simulink model "ingenuity_2023b"  (R2023b)
settings: Solver=VariableStepAuto  StartTime=0.0  StopTime=1000  FixedStep=0.001  RelTol=1e-3
values from neighbouring files (symbols this model uses):
  NACA2412 =     [CL_CD.mat]
undefined symbols (not defined in the file or in its folder): Actor, init
libraries: cstblocks x8, sim3dlib x7
settings Model: Creator=39351  LastModifiedBy=antor
settings OptimizationCC: ReuseModelBlockBuffer=off

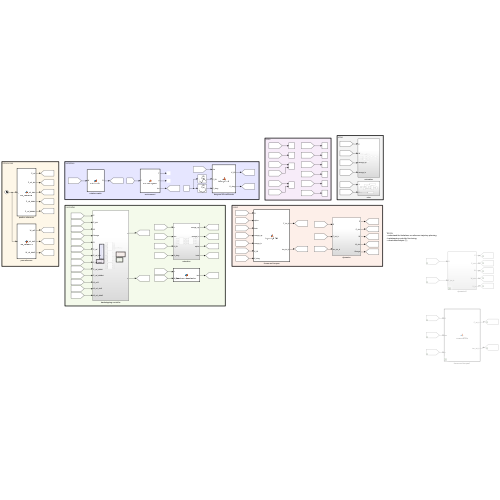
[thumbnail: Simulink's stored preview of the top-level diagram]
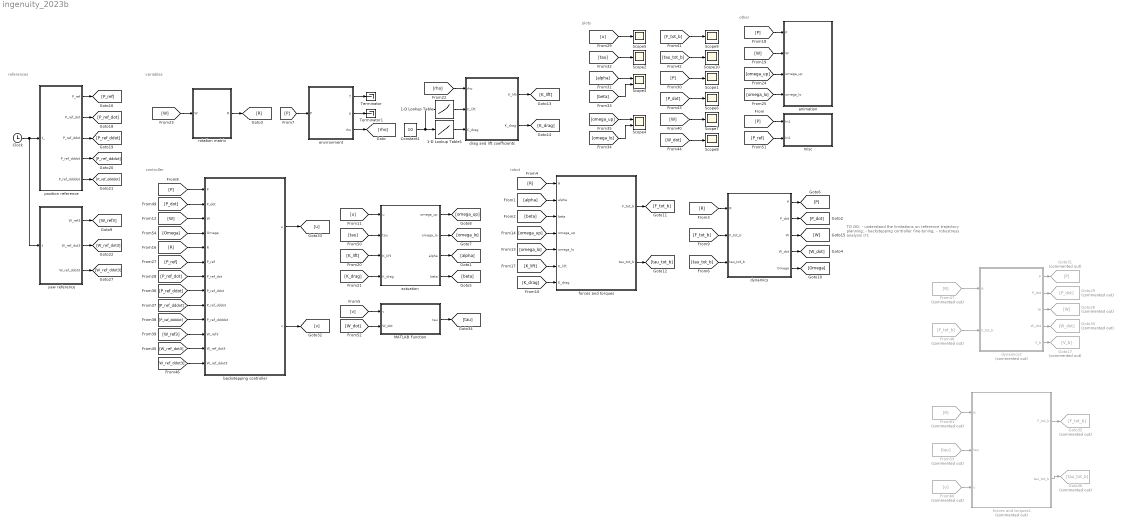
== system ingenuity_2023b ==
  note: TO DO:
      | - understand the limitations on reference trajectory planning;
      | - backstepping controller fine-tuning;
      | - robustness analysis (?);
  note: references
  note: other
  note: plots
  note: variables
  note: controller
  note: robot
  1-D Lookup Table : Lookup_n-D  NumberOfTableDimensions=1  BreakpointsForDimension1=NACA2412.CL(:,1)  Table=NACA2412.CL(:,2)  InternalRulePriority=Speed  RndMeth=Simplest
  1-D Lookup Table1 : Lookup_n-D  NumberOfTableDimensions=1  BreakpointsForDimension1=NACA2412.CD(:,1)  Table=NACA2412.CD(:,2)  InternalRulePriority=Speed  RndMeth=Simplest
  Clock : Clock
  Constant1 : Constant  Value=10
  From47 : From  Commented=on  GotoTag=R
  From48 : From  Commented=on  GotoTag=F_tot_b
  From53 : From  Commented=on  GotoTag=tau
  From60 : From  Commented=on  GotoTag=u
  From61 : From  Commented=on  GotoTag=R
  Goto17 : Goto  Commented=on  GotoTag=V_b
  Goto28 : Goto  Commented=on  GotoTag=W
  Goto29 : Goto  Commented=on  GotoTag=P_dot
  Goto30 : Goto  Commented=on  GotoTag=W_dot
  Goto31 : Goto  Commented=on  GotoTag=P
  Goto35 : Goto  Commented=on  GotoTag=F_tot_b
  Goto36 : Goto  Commented=on  GotoTag=tau_tot_b
  MATLAB Function : MATLAB Function  TreatAsAtomicUnit=on
  Scope{1..2,5..10} (8 alike) : Scope
  Scope3 : Scope  NumInputPorts=2
  Scope4 : Scope  NumInputPorts=2
  Terminator : Terminator
  Terminator1 : Terminator
  actuation : Subsystem
  animation : Subsystem
  backstepping controller : Subsystem
  drag and lift coefficients : MATLAB Function  TreatAsAtomicUnit=on
  dynamics : Subsystem
  dynamics2 : Subsystem  Commented=on
  environment : MATLAB Function  TreatAsAtomicUnit=on
  forces and torques : MATLAB Function  TreatAsAtomicUnit=on
  forces and torques1 : MATLAB Function  Commented=on  TreatAsAtomicUnit=on
  misc : Subsystem
  position reference : MATLAB Function  TreatAsAtomicUnit=on
  rotation matrix : MATLAB Function  TreatAsAtomicUnit=on
  yaw reference : MATLAB Function  TreatAsAtomicUnit=on
  wires:
  environment/1(T) -> Terminator/1
  environment/2(p) -> Terminator1/1
  environment/3(rho) -> [rho]
  [R] -> dynamics/1(R)
  dynamics/3(W) -> [W]
  [alpha] -> forces and torques/2(alpha)
  [beta] -> forces and torques/3(beta)
  [R] -> forces and torques/1(R)
  forces and torques/2(tau_tot_b) -> [tau_tot_b]
  forces and torques/1(F_tot_b) -> [F_tot_b]
  [F_tot_b] -> dynamics/2(F_tot_b)
  [tau_tot_b] -> dynamics/3(tau_tot_b)
  dynamics/4(W_dot) -> [W_dot]
  dynamics/1(P) -> [P]
  dynamics/2(P_dot) -> [P_dot]
  [omega_lo] -> forces and torques/5(omega_lo)
  [omega_up] -> forces and torques/4(omega_up)
  rotation matrix/1(R) -> [R]
  [W] -> rotation matrix/1(W)
  [K_lift] -> forces and torques/6(K_lift)
  [K_drag] -> forces and torques/7(K_drag)
  [rho] -> drag and lift coefficients/1(rho)
  drag and lift coefficients/1(K_lift) -> [K_lift]
  drag and lift coefficients/2(K_drag) -> [K_drag]
  1-D Lookup Table/1 -> drag and lift coefficients/2(C_lift)
  1-D Lookup Table1/1 -> drag and lift coefficients/3(C_drag)
  Constant1/1 -> 1-D Lookup Table1/1, 1-D Lookup Table/1
  [P] -> animation/1(P)
  [W] -> animation/2(W)
  [omega_up] -> animation/3(omega_up)
  [omega_lo] -> animation/4(omega_lo)
  [P] -> misc/1(In1)
  [P] -> Scope1/1
  [tau] -> Scope2/1
  [alpha] -> Scope3/1
  [beta] -> Scope3/2
  [omega_up] -> Scope4/1
  [omega_lo] -> Scope4/2
  [P] -> environment/1(P)
  position reference/1(P_ref) -> [P_ref]
  [u] -> Scope5/1
  position reference/2(P_ref_dot) -> [P_ref_dot]
  position reference/3(P_ref_ddot) -> [P_ref_ddot]
  [P_dot] -> Scope6/1
  [W] -> Scope7/1
  [W_dot] -> Scope8/1
  [F_tot_b] -> Scope9/1
  [tau_tot_b] -> Scope10/1
  [P_ref] -> misc/2(In2)
  position reference/4(P_ref_dddot) -> [P_ref_dddot]
  position reference/5(P_ref_ddddot) -> [P_ref_ddddot]
  yaw reference/2(W_ref_dot3) -> [W_ref_dot3]
  yaw reference/3(W_ref_ddot3) -> [W_ref_ddot3]
  Clock/1 -> yaw reference/1(t), position reference/1(t_)
  yaw reference/1(W_ref3) -> [W_ref3]
  [P] -> backstepping controller/1(P)
  [P_dot] -> backstepping controller/2(P_dot)
  [W] -> backstepping controller/3(W)
  [Omega] -> backstepping controller/4(Omega)
  [R] -> backstepping controller/5(R)
  [P_ref] -> backstepping controller/6(P_ref)
  [P_ref_dot] -> backstepping controller/7(P_ref_dot)
  [P_ref_ddot] -> backstepping controller/8(P_ref_ddot)
  [P_ref_dddot] -> backstepping controller/9(P_ref_dddot)
  [P_ref_ddddot] -> backstepping controller/10(P_ref_ddddot)
  [W_ref3] -> backstepping controller/11(W_ref3)
  [W_ref_dot3] -> backstepping controller/12(W_ref_dot3)
  [W_ref_ddot3] -> backstepping controller/13(W_ref_ddot3)
  dynamics2/5(V_b) -> Goto17/1
  dynamics2/2(P_dot) -> Goto29/1
  dynamics2/1(P) -> Goto31/1
  dynamics2/4(W_dot) -> Goto30/1
  dynamics2/3(W) -> Goto28/1
  From48/1 -> dynamics2/2(F_tot_b)
  From47/1 -> dynamics2/1(R)
  actuation/3(alpha) -> [alpha]
  [K_lift] -> actuation/3(K_lift)
  actuation/2(omega_lo) -> [omega_lo]
  [K_drag] -> actuation/4(K_drag)
  actuation/4(beta) -> [beta]
  actuation/1(omega_up) -> [omega_up]
  backstepping controller/2(v) -> [v]
  backstepping controller/1(u) -> [u]
  [v] -> MATLAB Function/1(v)
  [u] -> actuation/1(u)
  MATLAB Function/1(tau) -> [tau]
  [tau] -> actuation/2(tau)
  [W_dot] -> MATLAB Function/2(W_dot)
  From60/1 -> forces and torques1/3(u)
  From61/1 -> forces and torques1/1(R)
  forces and torques1/1(F_tot_b) -> Goto35/1
  From53/1 -> forces and torques1/2(tau)
  forces and torques1/2(tau_tot_b) -> Goto36/1
  dynamics/5(Omega) -> [Omega]

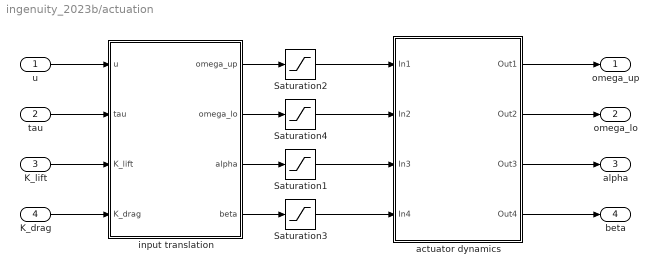
== system ingenuity_2023b/actuation ==
  u : Inport
  tau : Inport  Port=2
  K_lift : Inport  Port=3
  K_drag : Inport  Port=4
  Saturation1 : Saturate  UpperLimit=init.alpha_max  LowerLimit=-init.alpha_max  ZeroCross=off
  Saturation2 : Saturate  UpperLimit=init.omega_max  LowerLimit=0  ZeroCross=off
  Saturation3 : Saturate  UpperLimit=init.alpha_max  LowerLimit=-init.alpha_max  ZeroCross=off
  Saturation4 : Saturate  UpperLimit=init.omega_max  LowerLimit=0  ZeroCross=off
  actuator dynamics : Subsystem
  input translation : MATLAB Function  TreatAsAtomicUnit=on
  omega_up : Outport
  omega_lo : Outport  Port=2
  alpha : Outport  Port=3
  beta : Outport  Port=4
  wires:
  K_lift/1 -> input translation/3(K_lift)
  K_drag/1 -> input translation/4(K_drag)
  u/1 -> input translation/1(u)
  input translation/3(alpha) -> Saturation1/1
  input translation/4(beta) -> Saturation3/1
  tau/1 -> input translation/2(tau)
  input translation/1(omega_up) -> Saturation2/1
  Saturation2/1 -> actuator dynamics/1(In1)
  input translation/2(omega_lo) -> Saturation4/1
  Saturation1/1 -> actuator dynamics/3(In3)
  Saturation3/1 -> actuator dynamics/4(In4)
  actuator dynamics/1(Out1) -> omega_up/1
  actuator dynamics/2(Out2) -> omega_lo/1
  actuator dynamics/3(Out3) -> alpha/1
  actuator dynamics/4(Out4) -> beta/1
  Saturation4/1 -> actuator dynamics/2(In2)

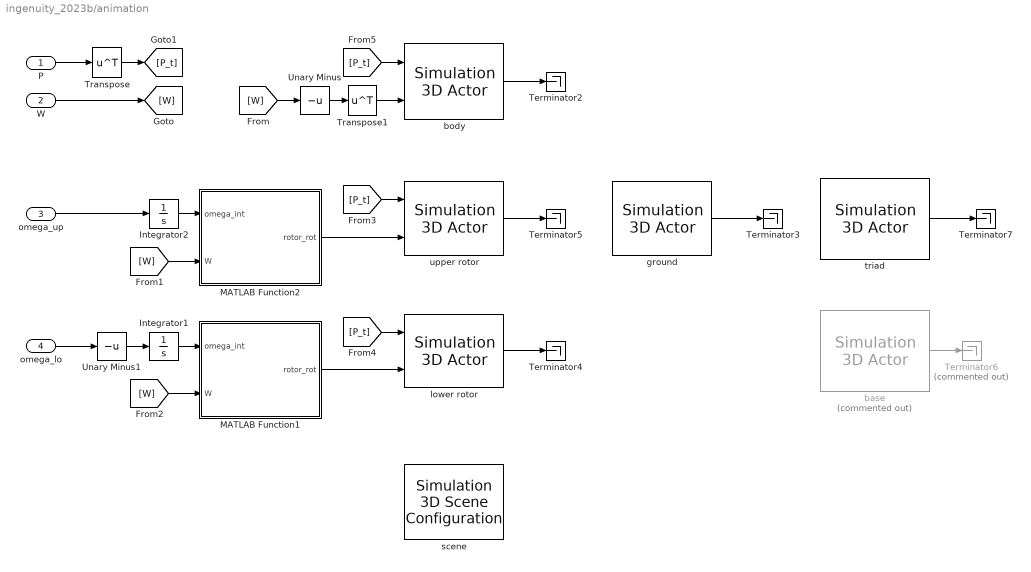
== system ingenuity_2023b/animation ==
  P : Inport
  W : Inport  Port=2
  omega_up : Inport  Port=3
  omega_lo : Inport  Port=4
  Integrator1 : Integrator  WrapState=on
  Integrator2 : Integrator  WrapState=on
  MATLAB Function1 : MATLAB Function  TreatAsAtomicUnit=on
  MATLAB Function2 : MATLAB Function  TreatAsAtomicUnit=on
  Terminator{2..5,7} (5 alike) : Terminator
  Terminator6 : Terminator  Commented=on
  Transpose : Math  Operator=transpose
  Transpose1 : Math  Operator=transpose
  Unary Minus : UnaryMinus
  Unary Minus1 : UnaryMinus
  base : sim3dlib/Simulation 3D Actor  Commented=on  ActorName=base  ParentName=Scene Origin  Operation=Create at setup  InitScriptText=Actor.createShape('box', [1 1 0.001]);  SampleTime=-1  Translation=single([0 0 0])  Rotation=single([0 0 0])  Scale=single([1 1 1])  aMode=5  ActorTag=base  ActorType=Sim3dActor  ID=C
      settings: LibrarySourceBlock=sl3dlib/Simulation 3D/Simulation 3D Actor
  body : sim3dlib/Simulation 3D Actor  ActorName=body  ParentName=Scene Origin  Operation=Create at setup  InitScriptText=|  SampleTime=-1  Translation=single([0 0 0])  Rotation=single([0 0 0])  Scale=single([1 1 1])  InputsText=body.Translation body.Rotation  aMode=5  ActorTag=body  ActorType=Sim3dActor  ID=C
      | % Actor.createShape('box', [0.5 0.5 0.1]);
      | Actor.Scale = [0.1 0.1 0.1];
      | Actor.Mobility = sim3d.utils.MobilityTypes.Movable;
      | % Actor.Gravity = true;
      | Actor.Shadows = true;
      | %Actor.Color = [0 0 0];
      settings: LibrarySourceBlock=sl3dlib/Simulation 3D/Simulation 3D Actor
  ground : sim3dlib/Simulation 3D Actor  ActorName=ground  ParentName=Scene Origin  Operation=Create at setup  InitScriptText=|  SampleTime=-1  Translation=single([0 0 0])  Rotation=single([0 0 0])  Scale=single([1 1 1])  aMode=5  ActorTag=ground  ActorType=Sim3dActor  ID=C
      | Actor.createShape('terrain', [1000 1000 0.001]);
      | Actor.PreciseContacts = true;
      | Actor.Color = [193, 68, 14]/255;
      settings: LibrarySourceBlock=sl3dlib/Simulation 3D/Simulation 3D Actor
  lower rotor : sim3dlib/Simulation 3D Actor  ActorName=lower_rotor  ParentName=Scene Origin  Operation=Create at setup  InitScriptText=|  SampleTime=-1  Translation=single([0 0 0])  Rotation=single([0 0 0])  Scale=single([1 1 1])  InputsText=lower_rotor.Translation lower_rotor.Rotation  aMode=5  ActorTag=lower_rotor  ActorType=Sim3dActor  ID=C
      | Actor.Mobility = sim3d.utils.MobilityTypes.Movable;
      | Actor.Shadows = true;
      | Actor.Scale = [0.1 0.1 0.1];
      | Actor.Color = [0 0 0];
      settings: LibrarySourceBlock=sl3dlib/Simulation 3D/Simulation 3D Actor
  scene : sim3dlib/Simulation 3D Scene Configuration  Priority=0  ProjectFormat=Default Scenes  SceneDesc=Empty scene  ProjectName=C:\Program Files\MATLAB\R2023b\toolbox\shared\sim3d_projects\automotive_project_windows\UE\WindowsNoEditor\VehicleSimulation.exe  ScenePath=/Game/Maps/HwStrght  EnableOpenDRIVE=off  vehTagList={'Custom';'Scene Origin';'Sim3dActor2';'Sim3dActor3';'body';'ground';'lower_rotor';'upper_rotor'}  vehTag=Scene Origin  FreeCameraInitialTranslation=[0, 0, 0]  FreeCameraDefaultInitialTranslation=[-6, 0, 2]  FreeCameraInitialRotation=[0, 0, 0]  FreeCameraDefaultInitialRotation=[0, -15, 0]  OpVisEn=off  Ts=0.02  EnableWindow=on  EnableRemoteAccess=off  EnableWeather=off  SunAltitude=40.0  SunAzimuth=90  clouds=10  wind=1  fog=9.0  rain=15.0  EnableGeospatial=off  OriginHeight=200  OriginLatitude=40.744652  OriginLongitude=-73.988864  MapStyle=Aerial  AdditionalAssetIDs=[]  UseAdvancedSunSky=off  SolarTime=11  TimeZone=-5  Day=21  Month=9  Year=2022  UseDaylightSavingTime=on  DSTStartDay=10  DSTStartMonth=3  DSTEndDay=3  DSTEndMonth=11  DSTSwitchHour=2  sensorTag=MainCamera1  sensorId=1  sensorName=MainCamera1  mountLoc=Origin  offsetFlag=off  tmountOffset=[0, 0, 0]  rmountOffset=[0, 0, 0]  HorizontalResolution=1280  VerticalResolution=720  HorizontalFOV=60  mountPoint=[0 0 0]  mountOrientation=[0 0 0]  aMode=5  ID=1  GeoTrigger=Inactive
      settings: LibrarySourceBlock=sl3dlib/Simulation 3D/Simulation 3D Scene Configuration
  triad : sim3dlib/Simulation 3D Actor  ActorName=triad  ParentName=Scene Origin  Operation=Create at setup  InitScriptText=|  SampleTime=-1  Translation=single([0 0 0])  Rotation=single([0 0 0])  Scale=single([1 1 1])  aMode=5  ActorTag=triad  ActorType=Sim3dActor  ID=C
      | Actor.Color = [1 0 0];
      | Actor.Scale = [0.003 0.003 0.003];
      settings: LibrarySourceBlock=sl3dlib/Simulation 3D/Simulation 3D Actor
  upper rotor : sim3dlib/Simulation 3D Actor  ActorName=upper_rotor  ParentName=Scene Origin  Operation=Create at setup  InitScriptText=|  SampleTime=-1  Translation=single([0 0 0])  Rotation=single([0 0 0])  Scale=single([1 1 1])  InputsText=upper_rotor.Translation upper_rotor.Rotation  aMode=5  ActorTag=upper_rotor  ActorType=Sim3dActor  ID=C
      | Actor.Mobility = sim3d.utils.MobilityTypes.Movable;
      | Actor.Shadows = true;
      | Actor.Scale = [0.1 0.1 0.1];
      | Actor.Color = [0 0 0];
      settings: LibrarySourceBlock=sl3dlib/Simulation 3D/Simulation 3D Actor
  wires:
  ground/1 -> Terminator3/1
  body/1 -> Terminator2/1
  upper rotor/1 -> Terminator5/1
  lower rotor/1 -> Terminator4/1
  P/1 -> Transpose/1
  Integrator2/1 -> MATLAB Function2/1(omega_int)
  Integrator1/1 -> MATLAB Function1/1(omega_int)
  Unary Minus/1 -> Transpose1/1
  Transpose1/1 -> body/2
  MATLAB Function2/1(rotor_rot) -> upper rotor/2
  omega_up/1 -> Integrator2/1
  omega_lo/1 -> Unary Minus1/1
  MATLAB Function1/1(rotor_rot) -> lower rotor/2
  Unary Minus1/1 -> Integrator1/1
  base/1 -> Terminator6/1
  W/1 -> [W]
  [W] -> Unary Minus/1
  [W] -> MATLAB Function2/2(W)
  [W] -> MATLAB Function1/2(W)
  Transpose/1 -> [P_t]
  [P_t] -> upper rotor/1
  [P_t] -> lower rotor/1
  [P_t] -> body/1
  triad/1 -> Terminator7/1

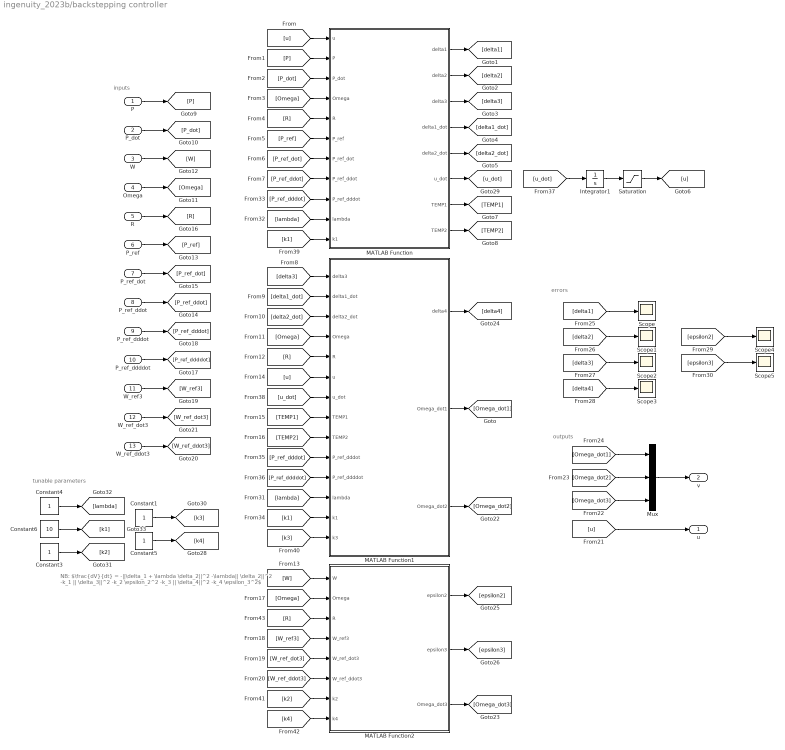
== system ingenuity_2023b/backstepping controller ==
  note: NB: $\frac{dV}{dt} = -||\delta_1 + \lambda \delta_2||^2 -\lambda|| \delta_2||^2 -k_1 || \delta_3||^2 -k_2 \epsilon_2^2 -k_3 || \delta_4||^2 -k_4 \epsilon_3^2$
  note: tunable parameters
  note: outputs
  note: inputs
  note: errors
  P : Inport
  P_dot : Inport  Port=2
  W : Inport  Port=3
  Omega : Inport  Port=4
  R : Inport  Port=5
  P_ref : Inport  Port=6
  P_ref_dot : Inport  Port=7
  P_ref_ddot : Inport  Port=8
  P_ref_dddot : Inport  Port=9
  P_ref_ddddot : Inport  Port=10
  W_ref3 : Inport  Port=11
  W_ref_dot3 : Inport  Port=12
  W_ref_ddot3 : Inport  Port=13
  Constant{1,3..5} (4 alike) : Constant
  Constant6 : Constant  Value=10
  Integrator1 : Integrator  InitialCondition=[0; 0; -init.F_grav_i(3)]
  MATLAB Function : MATLAB Function  TreatAsAtomicUnit=on
  MATLAB Function1 : MATLAB Function  TreatAsAtomicUnit=on
  MATLAB Function2 : MATLAB Function  TreatAsAtomicUnit=on
  Mux : Mux  Inputs=3
  Saturation : Saturate  UpperLimit=inf  LowerLimit=init.tol  ZeroCross=off
  Scope{,1..5} (6 alike) : Scope
  u : Outport
  v : Outport  Port=2
  wires:
  MATLAB Function/6(u_dot) -> [u_dot]
  MATLAB Function/1(delta1) -> [delta1]
  MATLAB Function/2(delta2) -> [delta2]
  MATLAB Function/3(delta3) -> [delta3]
  MATLAB Function/4(delta1_dot) -> [delta1_dot]
  MATLAB Function/5(delta2_dot) -> [delta2_dot]
  MATLAB Function/7(TEMP1) -> [TEMP1]
  MATLAB Function/8(TEMP2) -> [TEMP2]
  [u] -> MATLAB Function/1(u)
  P/1 -> [P]
  P_dot/1 -> [P_dot]
  W/1 -> [W]
  Omega/1 -> [Omega]
  R/1 -> [R]
  P_ref_ddot/1 -> [P_ref_ddot]
  P_ref_dot/1 -> [P_ref_dot]
  P_ref/1 -> [P_ref]
  P_ref_dddot/1 -> [P_ref_dddot]
  P_ref_ddddot/1 -> [P_ref_ddddot]
  [P] -> MATLAB Function/2(P)
  [P_dot] -> MATLAB Function/3(P_dot)
  [Omega] -> MATLAB Function/4(Omega)
  [R] -> MATLAB Function/5(R)
  [P_ref] -> MATLAB Function/6(P_ref)
  [P_ref_dot] -> MATLAB Function/7(P_ref_dot)
  [P_ref_ddot] -> MATLAB Function/8(P_ref_ddot)
  [delta3] -> MATLAB Function1/1(delta3)
  [delta1_dot] -> MATLAB Function1/2(delta1_dot)
  [delta2_dot] -> MATLAB Function1/3(delta2_dot)
  [Omega] -> MATLAB Function1/4(Omega)
  [R] -> MATLAB Function1/5(R)
  [W] -> MATLAB Function2/1(W)
  [u] -> MATLAB Function1/6(u)
  [TEMP1] -> MATLAB Function1/8(TEMP1)
  [TEMP2] -> MATLAB Function1/9(TEMP2)
  [Omega] -> MATLAB Function2/2(Omega)
  W_ref_ddot3/1 -> [W_ref_ddot3]
  W_ref_dot3/1 -> [W_ref_dot3]
  W_ref3/1 -> [W_ref3]
  [W_ref3] -> MATLAB Function2/4(W_ref3)
  [W_ref_dot3] -> MATLAB Function2/5(W_ref_dot3)
  [W_ref_ddot3] -> MATLAB Function2/6(W_ref_ddot3)
  [u] -> u/1
  MATLAB Function1/2(Omega_dot1) -> [Omega_dot1]
  MATLAB Function1/3(Omega_dot2) -> [Omega_dot2]
  MATLAB Function2/3(Omega_dot3) -> [Omega_dot3]
  [Omega_dot3] -> Mux/3
  [Omega_dot2] -> Mux/2
  [Omega_dot1] -> Mux/1
  MATLAB Function1/1(delta4) -> [delta4]
  MATLAB Function2/1(epsilon2) -> [epsilon2]
  MATLAB Function2/2(epsilon3) -> [epsilon3]
  [delta1] -> Scope/1
  [delta2] -> Scope1/1
  [delta3] -> Scope2/1
  [epsilon3] -> Scope5/1
  [delta4] -> Scope3/1
  [epsilon2] -> Scope4/1
  [k3] -> MATLAB Function1/14(k3)
  [lambda] -> MATLAB Function1/12(lambda)
  [lambda] -> MATLAB Function/10(lambda)
  [P_ref_dddot] -> MATLAB Function/9(P_ref_dddot)
  Constant5/1 -> [k4]
  [k1] -> MATLAB Function1/13(k1)
  [P_ref_dddot] -> MATLAB Function1/10(P_ref_dddot)
  [P_ref_ddddot] -> MATLAB Function1/11(P_ref_ddddot)
  Integrator1/1 -> Saturation/1
  [u_dot] -> Integrator1/1
  [u_dot] -> MATLAB Function1/7(u_dot)
  [k1] -> MATLAB Function/11(k1)
  Mux/1 -> v/1
  [k4] -> MATLAB Function2/8(k4)
  [k2] -> MATLAB Function2/7(k2)
  Constant3/1 -> [k2]
  Constant1/1 -> [k3]
  Constant6/1 -> [k1]
  Constant4/1 -> [lambda]
  [R] -> MATLAB Function2/3(R)
  Saturation/1 -> [u]

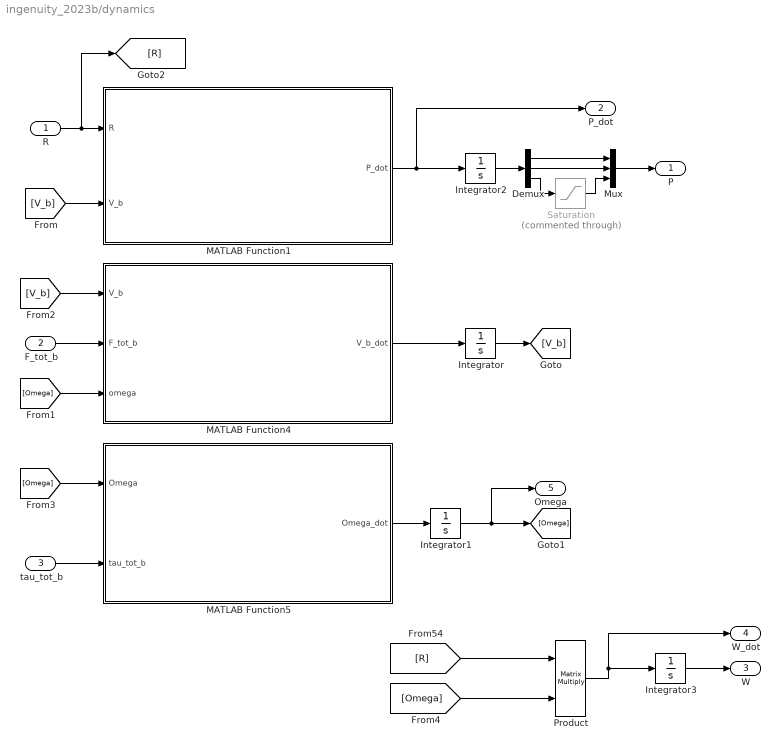
== system ingenuity_2023b/dynamics ==
  R : Inport
  F_tot_b : Inport  Port=2
  tau_tot_b : Inport  Port=3
  Demux : Demux  Outputs=3
  Integrator : Integrator  InitialCondition=[0 0 0]'
  Integrator1 : Integrator  InitialCondition=[0 0 0]'
  Integrator2 : Integrator  InitialCondition=[0 0 0]'
  Integrator3 : Integrator  InitialCondition=[0 0 0]'  WrapState=on
  MATLAB Function1 : MATLAB Function  TreatAsAtomicUnit=on
  MATLAB Function4 : MATLAB Function  TreatAsAtomicUnit=on
  MATLAB Function5 : MATLAB Function  TreatAsAtomicUnit=on
  Mux : Mux  Inputs=3
  Product : Product  Multiplication=Matrix(*)
  Saturation : Saturate  Commented=through  UpperLimit=inf  LowerLimit=-0.001
  P : Outport
  P_dot : Outport  Port=2
  W : Outport  Port=3
  W_dot : Outport  Port=4
  Omega : Outport  Port=5
  wires:
  R/1 -> [R], MATLAB Function1/1(R)
  MATLAB Function4/1(V_b_dot) -> Integrator/1
  MATLAB Function5/1(Omega_dot) -> Integrator1/1
  MATLAB Function1/1(P_dot) -> P_dot/1, Integrator2/1
  F_tot_b/1 -> MATLAB Function4/2(F_tot_b)
  tau_tot_b/1 -> MATLAB Function5/2(tau_tot_b)
  [V_b] -> MATLAB Function1/2(V_b)
  [Omega] -> MATLAB Function4/3(omega)
  [V_b] -> MATLAB Function4/1(V_b)
  [Omega] -> MATLAB Function5/1(Omega)
  Integrator/1 -> [V_b]
  Integrator2/1 -> Demux/1
  Integrator1/1 -> Omega/1, [Omega]
  Integrator3/1 -> W/1
  Mux/1 -> P/1
  Demux/1 -> Mux/1
  Demux/2 -> Mux/2
  Demux/3 -> Saturation/1
  Saturation/1 -> Mux/3
  [R] -> Product/1
  Product/1 -> Integrator3/1, W_dot/1
  [Omega] -> Product/2

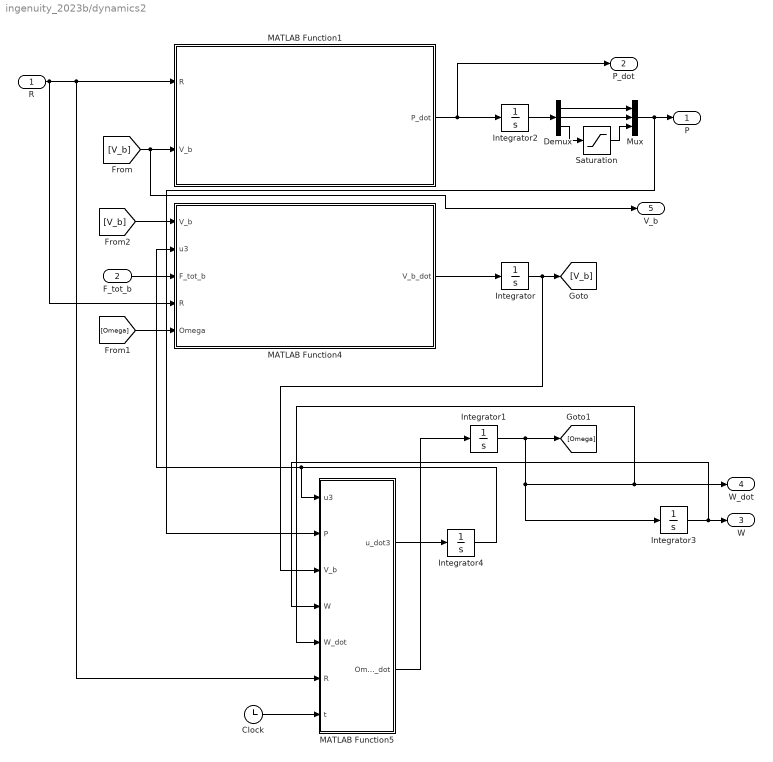
== system ingenuity_2023b/dynamics2 ==
  R : Inport
  F_tot_b : Inport  Port=2
  Clock : Clock
  Demux : Demux  Outputs=3
  Integrator : Integrator  InitialCondition=[0 0 0]'
  Integrator1 : Integrator  InitialCondition=[0 0 0]'
  Integrator2 : Integrator  InitialCondition=[0 0 0]'
  Integrator3 : Integrator  InitialCondition=[0 0 0]'  WrapState=on
  Integrator4 : Integrator  InitialCondition=-init.F_grav_i(3)
  MATLAB Function1 : MATLAB Function  TreatAsAtomicUnit=on
  MATLAB Function4 : MATLAB Function  TreatAsAtomicUnit=on
  MATLAB Function5 : MATLAB Function  TreatAsAtomicUnit=on
  Mux : Mux  Inputs=3
  Saturation : Saturate  UpperLimit=inf  LowerLimit=-0.001
  P : Outport
  P_dot : Outport  Port=2
  W : Outport  Port=3
  W_dot : Outport  Port=4
  V_b : Outport  Port=5
  wires:
  MATLAB Function4/1(V_b_dot) -> Integrator/1
  MATLAB Function1/1(P_dot) -> P_dot/1, Integrator2/1
  F_tot_b/1 -> MATLAB Function4/3(F_tot_b)
  [V_b] -> V_b/1, MATLAB Function1/2(V_b)
  [Omega] -> MATLAB Function4/5(Omega)
  [V_b] -> MATLAB Function4/1(V_b)
  Integrator/1 -> MATLAB Function5/3(V_b), [V_b]
  Integrator2/1 -> Demux/1
  Integrator1/1 -> [Omega], MATLAB Function5/5(W_dot), W_dot/1, Integrator3/1
  Integrator3/1 -> MATLAB Function5/4(W), W/1
  Mux/1 -> MATLAB Function5/2(P), P/1
  Demux/1 -> Mux/1
  Demux/2 -> Mux/2
  Demux/3 -> Saturation/1
  Saturation/1 -> Mux/3
  R/1 -> MATLAB Function4/4(R), MATLAB Function5/6(R), MATLAB Function1/1(R)
  MATLAB Function5/2(Omega_dot) -> Integrator1/1
  MATLAB Function5/1(u_dot3) -> Integrator4/1
  Integrator4/1 -> MATLAB Function5/1(u3), MATLAB Function4/2(u3)
  Clock/1 -> MATLAB Function5/7(t)

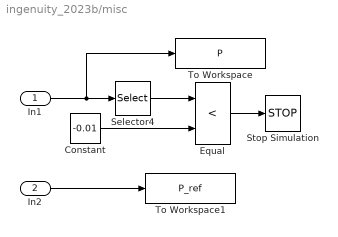
== system ingenuity_2023b/misc ==
  In1 : Inport
  In2 : Inport  Port=2
  Constant : Constant  Value=-0.01
  Equal : RelationalOperator  Operator=<  OutDataTypeStr=boolean  RndMeth=Simplest  InputSameDT=off
  Selector4 : Selector  InputPortWidth=3  IndexOptions=Index vector (dialog)  Indices=[3]  OutputSizes=1
  Stop Simulation : Stop
  To Workspace : ToWorkspace  VariableName=P  SaveFormat=Timeseries  SampleTime=-1
  To Workspace1 : ToWorkspace  VariableName=P_ref  SaveFormat=Timeseries  SampleTime=-1
  wires:
  Constant/1 -> Equal/2
  Selector4/1 -> Equal/1
  Equal/1 -> Stop Simulation/1
  In2/1 -> To Workspace1/1
  In1/1 -> To Workspace/1, Selector4/1

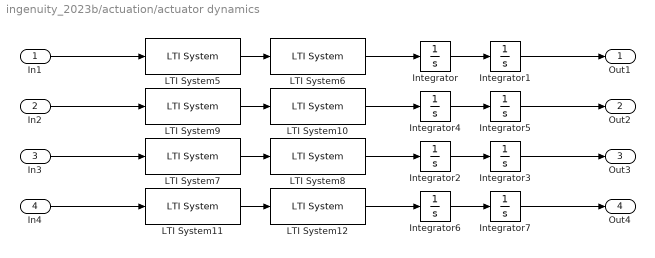
== system ingenuity_2023b/actuation/actuator dynamics ==
  In1 : Inport
  In2 : Inport  Port=2
  In3 : Inport  Port=3
  In4 : Inport  Port=4
  Integrator{,1..7} (8 alike) : Integrator
  LTI System{5..12} (8 alike) : cstblocks/LTI System  sys=tf([1 0] ,[0.001 1])  IC=[]  PadeOrder=0
  Out1 : Outport
  Out2 : Outport  Port=2
  Out3 : Outport  Port=3
  Out4 : Outport  Port=4
  wires:
  LTI System8/1 -> Integrator2/1
  Integrator1/1 -> Out1/1
  Integrator/1 -> Integrator1/1
  LTI System5/1 -> LTI System6/1
  In3/1 -> LTI System7/1
  In4/1 -> LTI System11/1
  Integrator6/1 -> Integrator7/1
  LTI System9/1 -> LTI System10/1
  Integrator7/1 -> Out4/1
  Integrator4/1 -> Integrator5/1
  LTI System12/1 -> Integrator6/1
  Integrator2/1 -> Integrator3/1
  LTI System10/1 -> Integrator4/1
  LTI System6/1 -> Integrator/1
  LTI System11/1 -> LTI System12/1
  Integrator5/1 -> Out2/1
  LTI System7/1 -> LTI System8/1
  Integrator3/1 -> Out3/1
  In2/1 -> LTI System9/1
  In1/1 -> LTI System5/1

== matlab function ingenuity_2023b/actuation/input translation ==
  data: omega_up output; omega_lo output; u input; tau input; K_lift input; K_drag input; alpha output; beta output; init parameter
function [omega_up, omega_lo, alpha, beta] = inputTranslation(u, tau, K_lift, K_drag, init)
    tol = 1e-5;
    
    d_com_lo = init.d_com_lo(3);
    d_com_up = init.d_com_up(3);

    tau3 = min(0.02*u(3)-tol, max(-0.02*u(3)+tol, tau(3)));
    
    omega_up = sqrt((u(3)+50*tau3)/(2*(K_lift - K_drag)));
    omega_lo = sqrt((u(3)-50*tau3)/(2*(K_lift - K_drag)));

    alpha = 2*tau(2)/((d_com_lo + d_com_up)*u(3) + 50*(d_com_up - d_com_lo)*tau3);
    beta = -2*tau(1)/((d_com_lo + d_com_up)*u(3) + 50*(d_com_up - d_com_lo)*tau3); 
end

== matlab function ingenuity_2023b/drag and lift coefficients ==
  data: rho input; C_lift input; C_drag input; K_lift output; K_drag output; init parameter
function [K_lift, K_drag] = liftDragCoeff(rho, C_lift, C_drag, init)
    c = init.c;
    r = init.r;

    K_lift = C_lift*c*rho*r^3/2;
    K_drag = C_drag*c*rho*r^3/2;
end

== matlab function ingenuity_2023b/animation/MATLAB Function1 ==
  data: omega_int input; W input; rotor_rot output
function rotor_rot = rotorRot(omega_int, W)
    rotz = [cos(omega_int) -sin(omega_int) 0; sin(omega_int) cos(omega_int) 0; 0 0 1];
    
    c1 = cos(W(1));
    s1 = sin(W(1));
    c2 = cos(W(2));
    s2 = sin(W(2));
    c3 = cos(W(3));
    s3 = sin(W(3));

    R = [c3*c2, c3*s2*s1 + s3*c1, -c3*s2*c1 + s3*s1;
         -s3*c2, -s3*s2*s1 + c3*c1, s3*s2*c1 + c3*s1;
         s2, -c2*s1, c2*c1];

    R_rotor = R*rotz;

    pitch = asin(-R_rotor(3,1));
    roll = atan2(R_rotor(3,2), R_rotor(3,3));
    yaw = atan2(R_rotor(2,1), R_rotor(1,1));


    rotor_rot = [roll, pitch, yaw];
end

== matlab function ingenuity_2023b/animation/MATLAB Function2 ==
  data: omega_int input; W input; rotor_rot output
function rotor_rot = rotorRot(omega_int, W)
    rotz = [cos(omega_int) -sin(omega_int) 0; sin(omega_int) cos(omega_int) 0; 0 0 1];
    
    c1 = cos(W(1));
    s1 = sin(W(1));
    c2 = cos(W(2));
    s2 = sin(W(2));
    c3 = cos(W(3));
    s3 = sin(W(3));

    R = [c3*c2, c3*s2*s1 + s3*c1, -c3*s2*c1 + s3*s1;
         -s3*c2, -s3*s2*s1 + c3*c1, s3*s2*c1 + c3*s1;
         s2, -c2*s1, c2*c1];

    R_rotor = R*rotz;

    pitch = asin(-R_rotor(3,1));
    roll = atan2(R_rotor(3,2), R_rotor(3,3));
    yaw = atan2(R_rotor(2,1), R_rotor(1,1));


    rotor_rot = [roll, pitch, yaw];
end

== matlab function ingenuity_2023b/position reference ==
  data: t_ input; P_ref output; P_ref_dot output; P_ref_ddot output; P_ref_dddot output; P_ref_ddddot output
function [P_ref, P_ref_dot, P_ref_ddot, P_ref_dddot, P_ref_ddddot] = pos_reference(t_)
    r = 3;
    d = 2;
    k = 5;

    t = mod(t_, 50);

    if(t > 30)
        P_ref = [0; 0; 0];
        P_ref_dot = [0; 0; 0];
        P_ref_ddot = [0; 0; 0];
        P_ref_dddot = [0; 0; 0];
        P_ref_ddddot = [0; 0; 0];
    else
        P_ref = [r*cos(t/d); r*sin(t/d); 1+t/k];
        P_ref_dot = [-r/d*sin(t/d); r/d*cos(t/d); 1/k];
        P_ref_ddot = [-r/d^2*cos(t/d); -r/d^2*sin(t/d); 0];
        P_ref_dddot = [0; 0; 0];
        P_ref_ddddot = [0; 0; 0];
    end

    % P_ref = [t^2/2; t^2/2; 1];
    % P_ref_dot = [t; t; 0];
    % P_ref_ddot = [1; 1; 0];
    % P_ref_dddot = [0; 0; 0];
    % P_ref_ddddot = [0; 0; 0];


end

== matlab function ingenuity_2023b/yaw reference ==
  data: t input; W_ref3 output; W_ref_dot3 output; W_ref_ddot3 output
function [W_ref3, W_ref_dot3, W_ref_ddot3] = yaw_reference(t)
    W_ref3 = 0;
    W_ref_dot3 = 0;
    W_ref_ddot3 = 0;
end

== matlab function ingenuity_2023b/backstepping controller/MATLAB Function ==
  data: u input; delta1 output; P input; P_dot input; Omega input; R input; P_ref input; P_ref_dot input; P_ref_ddot input; P_ref_dddot input; lambda input; k1 input; delta2 output; delta3 output; delta1_dot output; delta2_dot output; u_dot output; TEMP1 output; init parameter; TEMP2 output
function [delta1, delta2, delta3, delta1_dot, delta2_dot, u_dot, TEMP1, TEMP2] = liftControl(u, P, P_dot, ...
    Omega, R, P_ref, P_ref_dot, P_ref_ddot, P_ref_dddot, lambda, k1, init)

    m = init.m;
    F_grav_i = init.F_grav_i;

    F = R.'*F_grav_i +u;
    V_b = R.'*P_dot;

    delta1 = R.'*(P_ref-P);
    delta2 = R.'*P_ref_dot -V_b;
    delta1_dot = -cross(Omega, delta1) +delta2;
    delta2_dot = -cross(Omega, delta2) +R.'*P_ref_ddot -F/m;

    lambda_F_over_m_des = delta1 +(lambda +2)*delta2 +lambda*R.'*P_ref_ddot;
    delta3 = lambda_F_over_m_des -lambda/m*F;
    TEMP1 = (lambda+2)/lambda*delta3 -(lambda+2)/lambda*delta1 -(lambda^2+3*lambda+4)/lambda*delta2 +lambda*R.'*P_ref_dddot;
    TEMP2 = TEMP1 +(delta1 +lambda*delta2) +k1*delta3;
    u_dot3 = [0 0 1]*m/lambda*TEMP2;
    u_dot = [0; 0; u_dot3];
end

== matlab function ingenuity_2023b/backstepping controller/MATLAB Function1 ==
  data: delta3 input; delta1_dot input; delta2_dot input; Omega input; R input; u input; u_dot input; TEMP1 input; TEMP2 input; P_ref_dddot input; P_ref_ddddot input; lambda input; k1 input; k3 input; delta4 output; Omega_dot1 output; init parameter; Omega_dot2 output
function [delta4, Omega_dot1, Omega_dot2] = rollPitchControl(delta3, delta1_dot, ...
    delta2_dot, Omega, R, u, u_dot, TEMP1, TEMP2, P_ref_dddot, P_ref_ddddot, lambda, k1, k3, init)

    m = init.m;

    u3 = u(3);
    
    delta3_dot = -cross(Omega, delta3) -lambda/m*cross(Omega, u) +TEMP1 -lambda/m*u_dot;

    lambda_cross_W_dot_u_over_m_des = [1 0 0; 0 1 0; 0 0 0]*TEMP2;
    lambda_cross_W_dot_u_over_m_des_dot = [1 0 0; 0 1 0; 0 0 0]*(((lambda+2)/lambda +k1)*delta3_dot ...
        -((lambda+2)/lambda -1)*delta1_dot -((lambda^2+3*lambda+4)/lambda -lambda)*delta2_dot ...
        +lambda*R.'*P_ref_ddddot -lambda*cross(Omega, R.'*P_ref_dddot));
    delta4 = lambda_cross_W_dot_u_over_m_des -lambda/m*cross(Omega, u);
    TEMP3 = lambda_cross_W_dot_u_over_m_des_dot -lambda/m*cross(Omega, u_dot) +delta3 +k3*delta4;

    Omega_dot1 = -m/(lambda*u3)*[0 1 0]*TEMP3;
    Omega_dot2 = m/(lambda*u3)*[1 0 0]*TEMP3;
end

== matlab function ingenuity_2023b/backstepping controller/MATLAB Function2 ==
  data: W input; Omega input; R input; W_ref3 input; W_ref_dot3 input; W_ref_ddot3 input; k2 input; epsilon2 output; epsilon3 output; k4 input; Omega_dot3 output
function [epsilon2, epsilon3, Omega_dot3] = yawControl(W, Omega, R, W_ref3, W_ref_dot3 , W_ref_ddot3, k2, k4)
    W3 = W(3);

    W_dot = R*Omega;
    W_dot3 = W_dot(3);
    
    epsilon2 = W_ref3 -W3;
    W_dot3_virt = W_ref_dot3 +k2*epsilon2;

    epsilon3 = W_dot3_virt -W_dot3;

    W_ddot3 = (W_ref_ddot3 +k2*(W_ref_dot3 -W_dot3) +epsilon2 +k4*epsilon3);
    % Omega_dot3 = W_ddot3;

    Omega_dot3 = [0 0 1]*R.'*(W_ddot3 -cross(Omega, R*Omega));

    % M = [-sin(W2), 0, 1; cos(W2)*sin(W1), cos(W1), 0; cos(W2)*cos(W1), -sin(W1), 0];
    % M_dot = [-cos(W2)*W_dot2, 0, 1; 
    %     -sin(W2)*W_dot2*sin(W1)+cos(W2)*cos(W1)*W_dot1, -sin(W1)*W_dot1, 0; 
    %     -sin(W2)*W_dot2*cos(W1)-cos(W2)*sin(W1)*W_dot1, -cos(W1)*W_dot1, 0];

    % Omega_dot3 = cos(W2)/cos(W1)*(W_ddot3 + [0 0 1]*(M\(M_dot*(M\Omega))) -sin(W(1))/cos(W(2))*Omega_dot2);
end

== matlab function ingenuity_2023b/dynamics2/MATLAB Function1 ==
  data: R input; P_dot output; V_b input
function P_dot = positionDynamics(R, V_b)
    % positionDynamics calculates the derivative of position in the inertial frame
    P_dot = R*V_b;
end

== matlab function ingenuity_2023b/dynamics2/MATLAB Function4 ==
  data: V_b input; u3 input; F_tot_b input; R input; Omega input; V_b_dot output; init parameter
function V_b_dot = velocityDynamics(V_b, u3, F_tot_b, R, Omega,init)
    % velocityDynamics calculates the derivative of velocity in the body frame
    % Neglecting external force Fe, the cross product term accounts for the Coriolis effect
    F_grav_i = init.F_grav_i;
    u = [0; 0; u3];
    F_tot_b = R.'*F_grav_i +u;
    V_b_dot = F_tot_b/init.m - cross(Omega, V_b);
end

== matlab function ingenuity_2023b/dynamics2/MATLAB Function5 ==
  data: u_dot3 output; u3 input; P input; V_b input; W input; W_dot input; R input; t input; Omega_dot output; init parameter
function [u_dot3, Omega_dot] = fcn(u3, P, V_b, W, W_dot, R, t, init)
    m = init.m;
    F_grav_i = init.F_grav_i;

    r=10;
    d=30;
    k = 1000;

    P_des=[r*cos(t/d) ; r*sin(t/d) ; 1+t/k];
    P_dot_des=[-r/d*sin(t/d);r/d*cos(t/d);1/k];
    P_ddot_des=[-r/d^2*cos(t/d); -r/d^2*sin(t/d); 0];
    % P_des = [t^2/2; t^2/2; 1];
    % P_dot_des = [t; t; 0];
    % P_ddot_des = [1; 1; 0];
    P_dddot_des = [0; 0; 0];
    P_ddddot_des = [0; 0; 0];
    W_des3 = 0;
    W_dot_des3 = 0;
    W_ddot_des3 = 0;

    lambda = 1;
    k1 = 1;
    k2 = 1;
    k3 = 1;
    k4 = 1;

    W_dot3 = W_dot(3);
    W3 = W(3);
    u = [0; 0; u3];

    F = R.'*F_grav_i +u;

    delta1 = R.'*(P_des-P);
    delta2 = R.'*P_dot_des -V_b;
    delta1_dot = -cross(W_dot, delta1) +delta2;
    delta2_dot = -cross(W_dot, delta2) +R.'*P_ddot_des -R.'*F_grav_i/m -u/m;

    lambda_F_over_m_virt = delta1 +(lambda +2)*delta2 +lambda*R.'*P_ddot_des;
    delta3 = lambda_F_over_m_virt -lambda/m*F;
    A = (lambda+2)/lambda*delta3 -(lambda+2)/lambda*delta1 -(lambda^2+3*lambda+4)/lambda*delta2 +lambda*R.'*P_dddot_des;
    B = A +(delta1 +lambda*delta2) +k1*delta3;
    u_dot3 = [0 0 1]*m/lambda*B;
    u_dot = [0; 0; u_dot3];
    delta3_dot = -cross(W_dot, delta3) -lambda/m*cross(W_dot, u) +A -lambda/m*u_dot;
    epsilon2 = W_des3 -W3;
    W_dot3_virt = W_dot_des3 +k2*epsilon2;

    lambda_cross_W_dot_u_over_m_virt = [1 0 0; 0 1 0; 0 0 0]*B;
    lambda_cross_W_dot_u_over_m_virt_dot = [1 0 0; 0 1 0; 0 0 0]*(((lambda+2)/lambda +k1)*delta3_dot ...
        -((lambda+2)/lambda -1)*delta1_dot -((lambda^2+3*lambda+4)/lambda -lambda)*delta2_dot +lambda*R.'*P_ddddot_des -lambda*cross(W_dot, R.'*P_dddot_des));
    delta4 = lambda_cross_W_dot_u_over_m_virt -lambda/m*cross(W_dot, u);
    epsilon3 = W_dot3_virt -W_dot3;
    C = lambda_cross_W_dot_u_over_m_virt_dot -lambda/m*cross(W_dot, u_dot) +delta3 +k3*delta4;

    Omega_dot1 = -m/(lambda*u3)*[0 1 0]*C;
    Omega_dot2 = m/(lambda*u3)*[1 0 0]*C;
    % Omega_dot1 = 0;
    % Omega_dot2 = 0;
    Omega_dot3 = W_ddot_des3 +k2*(W_dot_des3 -W_dot3) +epsilon2 +k4*epsilon3;

    Omega_dot = [Omega_dot1; Omega_dot2; Omega_dot3];
end

== matlab function ingenuity_2023b/MATLAB Function ==
  data: v input; W_dot input; tau output; init parameter
function tau = feedbackLinearization(v, W_dot, init)
    I = init.I;
    tau = I*v + cross(W_dot, I*W_dot);
end

== matlab function ingenuity_2023b/forces and torques1 ==
  data: F_tot_b output; R input; tau input; u input; tau_tot_b output; init parameter
function [F_tot_b, tau_tot_b] = ingenuityEOM(R, tau, u, init)
    % Gravitational force in inertial frame
    F_grav_i = init.F_grav_i;

    tau_ac= 0;
    F_ac= 0;

    % Total force in body frame
    F_tot_b = u + R.'*F_grav_i + F_ac;
    
    % Total torque in body frame
    tau_tot_b = tau + tau_ac;

    % Other external unknown forces and torques are omitted
end

== matlab function ingenuity_2023b/forces and torques ==
  data: F_tot_b output; R input; alpha input; beta input; omega_up input; omega_lo input; tau_tot_b output; init parameter; K_lift input; K_drag input
function [F_tot_b, tau_tot_b] = ingenuityEOM(R, alpha, beta, omega_up, omega_lo, init, K_lift, K_drag)
    % Gravitational force in inertial frame
    F_grav_i = init.F_grav_i;
    d_com_up = init.d_com_up;
    d_com_lo = init.d_com_lo;
    
    % Thrust direction matrix T(alpha, beta)
    gamma = atan(sqrt(tan(alpha)^2 + tan(beta)^2));
    T = [tan(alpha)*cos(gamma); tan(beta)*cos(gamma); cos(gamma)];
    T = [alpha; beta; 1];

    % T = 1/sqrt(1-sin(alpha)^2*sin(beta)^2)*[sin(alpha)*cos(beta); sin(beta)*cos(alpha); cos(alpha)*cos(beta)];
    
    norm_F_up_b = abs(K_lift-K_drag)*omega_up^2;
    norm_F_lo_b = abs(K_lift-K_drag)*omega_lo^2;

    % Total lift force in body frame
    F_up_b = T*norm_F_up_b*sign(K_lift-K_drag);
    F_lo_b = T*norm_F_lo_b*sign(K_lift-K_drag);
    
    % Torques
    tau_lo = cross(d_com_lo, F_lo_b); % Torque due to lower rotor
    tau_up = cross(d_com_up, F_up_b); % Torque due to upper rotor
    
    % Reaction torques in body frame
    Q_lo = 0.02*norm_F_lo_b;
    Q_up = 0.02*norm_F_up_b;
    tau_react_b = [0; 0; Q_up-Q_lo];
    
    % Actuation coupling forces and torques
    % Gf=[0 -init.d_com_lo(3) 0;
    %     init.d_com_lo(3) 0 0;
    %     0 0 0];  
    G_for = zeros(3,3);
    
    % Gt=[0 1/init.d_com_lo(3) 0;
    %     -1/init.d_com_lo(3) 0 0;
    %     0 0 0];
    G_tor = zeros(3,3);

    F=F_lo_b+F_up_b;
    tau=tau_lo+tau_up+tau_react_b;

    tau_ac= G_for*F;
    F_ac= G_tor*tau;

    % Total force in body frame
    F_tot_b = F + R.'*F_grav_i + F_ac;
    
    % Total torque in body frame
    tau_tot_b = tau + tau_ac;

    % Other external unknown forces and torques are omitted
end

== matlab function ingenuity_2023b/environment ==
  data: P input; T output; p output; rho output
function [T, p, rho] = marsAtmosphere(P)
    % marsAtmosphere calculates the temperature, pressure, and density on Mars
    % as a function of altitude h (in meters).
    % Constants for pressure calculation in SI units
    p0 = 0.699; % Baseline pressure in K-Pa
    T0 = 273.1; % Reference temperature in Kelvin for density calculation

    h = P(3);
    
    if h > 7000
        % For altitudes above 7000 meters
        T = -23.4 - 0.00222 * h;
        p = p0 * exp(-0.00009 * h);
    else
        % For altitudes at or below 7000 meters
        T = -31 - 0.000998 * h;
        p = p0 * exp(-0.00009 * h);
    end
    
    % Convert temperature from Celsius to Kelvin for density calculation
    T_Kelvin = T + T0;
    
    % Calculate the density using the provided formula
    rho = p / (0.1921 * (T_Kelvin));
end

== matlab function ingenuity_2023b/rotation matrix ==
  data: W input; R output
function R  = rotationMat(W)
    c1 = cos(W(1));
    s1 = sin(W(1));
    c2 = cos(W(2));
    s2 = sin(W(2));
    c3 = cos(W(3));
    s3 = sin(W(3));

    R = [c3*c2, c3*s2*s1 - s3*c1, c3*s2*c1 + s3*s1;
         s3*c2, s3*s2*s1 + c3*c1, s3*s2*c1 - c3*s1;
         -s2, c2*s1, c2*c1];
end

== matlab function ingenuity_2023b/dynamics/MATLAB Function1 ==
  data: R input; P_dot output; V_b input
function P_dot = positionDynamics(R, V_b)
    % positionDynamics calculates the derivative of position in the inertial frame
    P_dot = R*V_b;
end

== matlab function ingenuity_2023b/dynamics/MATLAB Function4 ==
  data: V_b input; F_tot_b input; omega input; V_b_dot output; init parameter
function V_b_dot = velocityDynamics(V_b, F_tot_b, omega,init)
    % velocityDynamics calculates the derivative of velocity in the body frame
    % Neglecting external force Fe, the cross product term accounts for the Coriolis effect
    V_b_dot = F_tot_b/init.m - cross(omega, V_b);
end

== matlab function ingenuity_2023b/dynamics/MATLAB Function5 ==
  data: Omega input; tau_tot_b input; Omega_dot output; init parameter
function Omega_dot = angularVelocityDynamics(Omega, tau_tot_b, init)
    % angularVelocityDynamics calculates the derivative of angular velocity in the body frame
    % Neglecting external torque tau_e, the cross product term represents the gyroscopic effect
    Omega_dot = init.I\(tau_tot_b - cross(Omega, init.I*Omega));
end
